simulink model "player_ball_7_8players3_2_withemotion"  (R2021b)
settings: Solver=VariableStepAuto  StartTime=0.0  StopTime=300  RelTol=1e-3
model workspace (MAT data in the model file):
  trailfuzzy = 'trailfuzzy.fis'
values from neighbouring files (symbols this model uses):
  initBallPos = fieldCenter    [robotSoccerParams.m]
  robotDetectorMaxHits = 5    [robotSoccerParams.m]
  sampleTime = 0.05    [robotSoccerParams.m]
undefined symbols (not defined in the file or in its folder): DiscIntNeverNeededParam
libraries: mobileRoboticsLib x38, dspindex x12, fuzblock x9
(part 3 of 3)

== matlab function player_ball_7_8players3_2_withemotion/MATLAB Function12 ==
  data: Morale1 input; Morale output; Agg output; attack output; defense output; interception output; posession output; Agg1 input; attack1 input; defense1 input; team1_score input; team2_score input; goalscored input
function [Morale, Agg, attack, defense, interception, posession]= fcn(Morale1, Agg1, attack1, defense1,team1_score, team2_score,goalscored)
%emotions
Morale = Morale1;
Agg = Agg1;
attack = attack1;
defense = defense1;




score_diff =  -team1_score + team2_score
if goalscored == 1
    if score_diff > 0
        Agg = Agg - 0.1;
        Morale = -0.021*(Agg^5) + (0.2908)*(Agg^5) - 1.3933 * (Agg^3) + (2.375) * (Agg^2) - 0.8426*Agg + 4.1552;
        attack = attack + Agg/2;
        defense = defense + Agg/2;
     
    
    elseif score_diff < 0
        Agg = Agg + 0.1
        Morale = -0.021*(Agg^5) + (0.2908)*(Agg^5) - 1.3933 * (Agg^3) + (2.375) * (Agg^2) - 0.8426*Agg + 4.1552;
        attack = attack - Agg/2;
        defense = defense - Agg/2;
       


    end
end
pp = (attack + defense)*Morale + Agg;
ratio_a = 0.15;
ratio_b = 1 - ratio_a;


interception = ratio_a*pp;
posession = ratio_b*pp;

== matlab function player_ball_7_8players3_2_withemotion/MATLAB Function13 ==
  data: u input; angle output; range output
function [angle,range]= fcn(u)
a = u(1,:);
b = u(2,:);
c = u(3,:);
d = u(4,:);
e = u(5,:);

    if a(3) ==1
        angle = a(2);
        range = a(1);
      
    elseif b(3) ==1
        angle = b(2);
        range = b(1);
    elseif c(3) ==1
        angle = c(2);
        range = c(1);
    elseif d(3)==1
        angle = d(2);
        range = d(1);
    else
        angle = 3.14;
        range = 35;
    end
end

== matlab function player_ball_7_8players3_2_withemotion/MATLAB Function14 ==
  data: u input; angle output; range output
function [angle,range]= fcn(u)
a = u(1,:);
b = u(2,:);
c = u(3,:);
d = u(4,:);
e = u(5,:);

    if a(3) ==1
        angle = a(2);
        range = a(1);
      
    elseif b(3) ==1
        angle = b(2);
        range = b(1);
    elseif c(3) ==1
        angle = c(2);
        range = c(1);
    elseif d(3)==1
        angle = d(2);
        range = d(1);
    else
        angle = 3.14;
        range = 35;
    end
end
